simulink model "figure_3_speed_load_control_block"  (R2021a)
settings: Solver=VariableStepAuto  StartTime=0.0  StopTime=10.0  RelTol=1e-3
model workspace (MAT data in the model file):
  C = 2
  R = 1
  Tb = Simulink.Parameter
  Tb.DataType = 'auto'
  Tb.Dimensions = [0 0]
  Tcd = Simulink.Parameter
  Tcd.DataType = 'auto'
  Tcd.Dimensions = [0 0]
  Tg = Simulink.Parameter
  Tg.DataType = 'auto'
  Tg.Dimensions = [0 0]
  Tl = Simulink.Parameter
  Tl.DataType = 'auto'
  Tl.Dimensions = [0 0]
  Tm = Simulink.Parameter
  Tm.DataType = 'auto'
  Tm.Dimensions = [0 0]
settings Model: Creator=Souvik Datta  LastModifiedBy=Souvik Datta
settings SolverCC: AlgebraicLoopSolver=TrustRegion
settings DebuggingCC: SFMachineParentedDataDiag=warning

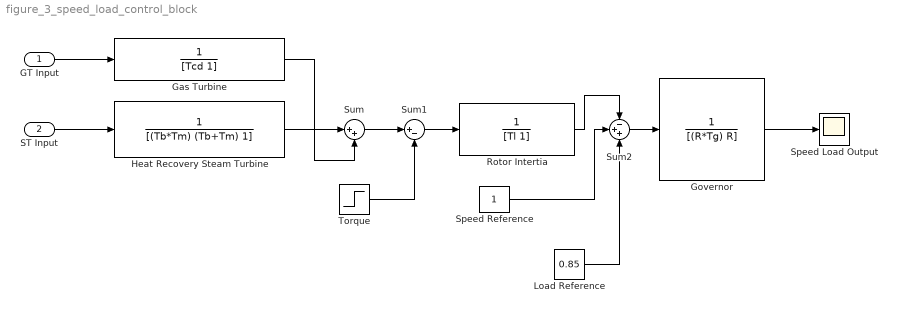
== system figure_3_speed_load_control_block ==
  GT Input : Inport
  ST Input : Inport  Port=2
  Gas Turbine : TransferFcn  Denominator=[Tcd 1]
  Governor : TransferFcn  Denominator=[(R*Tg) R]
  Heat Recovery Steam Turbine : TransferFcn  Denominator=[(Tb*Tm) (Tb+Tm) 1]
  Load Reference : Constant  Value=0.85
  Rotor Intertia : TransferFcn  Denominator=[Tl 1]
  Speed Load Output : Scope
  Speed Reference : Constant
  Sum : Sum  Inputs=|++
  Sum1 : Sum  Inputs=|+-
  Sum2 : Sum  Inputs=-++
  Torque : Step  SampleTime=0
  wires:
  ST Input/1 -> Heat Recovery Steam Turbine/1
  Heat Recovery Steam Turbine/1 -> Sum/1
  GT Input/1 -> Gas Turbine/1
  Gas Turbine/1 -> Sum/2
  Sum/1 -> Sum1/1
  Torque/1 -> Sum1/2
  Sum1/1 -> Rotor Intertia/1
  Sum2/1 -> Governor/1
  Rotor Intertia/1 -> Sum2/1
  Speed Reference/1 -> Sum2/2
  Load Reference/1 -> Sum2/3
  Governor/1 -> Speed Load Output/1
